simulink model "am_ssb"  (R2014b)
settings: Solver=ode45  StartTime=0.0  StopTime=0.06  RelTol=1e-3
PreLoadFcn:
  | %%%%%%%%%%%%%%%%%%%%%%%%%%%%%%%%%%%%%%%%%%%%%%%%%%%%%%%%%%%%%%%%%%%%%%%%%%%
  | % check to see if Simulink library folder is missing from the MATLAB path %
  | %%%%%%%%%%%%%%%%%%%%%%%%%%%%%%%%%%%%%%%%%%%%%%%%%%%%%%%%%%%%%%%%%%%%%%%%%%%
  | if isempty(strfind(path, 'rtlsdr_book_library'))
  | 
  |     % create error window
  |     fig_error = figure(...
  |         'Name', 'Error: RTL-SDR Book Library',...
  |         'Toolbar','none',...
  |         'MenuBar','none',...
  |         'NumberTitle','off',...
  |         'Resize','off',...
  |         'WindowStyle','modal');
  |     fig_error.Position(3) = 600;
  |     fig_error.Position(4) = 150;
  |     fig_axes = axes(...
  |         'Parent',fig_error,...
  |         'Position',[0,0,1,1],...
  |         'visible','off');
  |     % error message
  |     t_title = text(.05,.8,...
  |         'MISSING DIRECTORIES',...
  |         'FontSize',11.5);
  |     t_body = text(.075,.6,...
  |         [{'Simulink cannot find the  \it{<root>}\rm / \it{rtlsdr\_book\_library}\rm  folder in the \it{MATLAB Path}\rm.'},...
  |         {'Please set the MATLAB path following the instructions given in Exercise 2.4.'}],...
  |         'FontSize',10.5);
  |     % buttons
  |     btn_path = uicontrol(...
  |         'Parent',fig_error,...
  |         'String','Set Path Now',...
  |         'FontSize',10,...
  |         'Callback', 'pathtool; close(fig_error);',...
  |         'Position', [fig_error.Position(3)/2-210, 30, 200, 30]);
  |     btn_abort = uicontrol(...
  |         'Parent',fig_error,...
  |         'String','No thanks',...
  |         'FontSize',10,...
  |         'Callback', 'close(fig_error); abort=1;',...
  |         'Position', [fig_error.Position(3)/2+10, 30, 200, 30]);
  | 
  |     % pause to allow user to interact with error box
  |     uiwait(fig_error);
  | 
  |     % abort simulation
  |     try
  |         if abort==1
  |             set_param(gcs, 'SimulationCommand', 'stop');
  |         end
  |     end
  | 
  |     % if user has set path, allow diagram to be updated
  |     if ~exist('abort','var')
  |         % create error window
  |         fig_update = figure(...
  |             'Name', 'Update Diagram',...
  |             'Toolbar','none',...
  |             'MenuBar','none',...
  |             'NumberTitle','off',...
  |             'Resize','off');
  |         fig_update.Position(3) = 400;
  |         fig_update.Position(4) = 120;
  |         fig_axes = axes(...
  |             'Parent',fig_update,...
  |             'Position',[0,0,1,1],...
  |             'visible','off');
  |         % instruction message
  |         t_body = text(.075,.7,...
  |             'Once you have set the path, update the block diagram',...
  |             'FontSize',10.5);
  |         % button
  |         btn_update = uicontrol(...
  |             'Parent',fig_update,...
  |             'String','Update Block Diagram',...
  |             'FontSize',10,...
  |             'Callback', 'set_param(gcs,''SimulationCommand'',''update''); close(gcf)',...
  |             'Position', [fig_update.Position(3)/2-100, 30, 200, 30]);
  |     end
  | 
  |     % clear error components
  |     clear('fig_error','fig_update','fig_axes','t_title','t_body','btn_path','btn_abort','btn_update','abort');
  | 
  | end
  | %%%%%%%%%%%%%%%%%%%%%%%%%%%%%%%%%%%%%%%%%%%%%%%%%%%%%%%%%%%%%%%%%%%%%%%%%%%
PostLoadFcn:
  | fs  = 200e3;
  | 
  | single.Ai = 8;
  | single.fi = 3e3;
  | single.ph = 0;
  | 
  | bband1.Ai = 1;
  | bband1.fi = 2e3;
  | bband1.ph = pi/2;
  | 
  | bband2.Ai = 3;
  | bband2.fi = 3e3;
  | bband2.ph = 0;
  | 
  | bband3.Ai = 2;
  | bband3.fi = 4e3;
  | bband3.ph = pi/4;
  | 
  | bband4.Ai = 5;
  | bband4.fi = 5e3;
  | bband4.ph = pi/3;
  | 
  | carrier.Ac = 1;
  | carrier.fc = 15e3;
  | carrier.ph = pi/2;
undefined symbols (not defined in the file): fdesignblkfcn, gcbh, startfcn_spectrum_analyzer, startfcn_time_scope
libraries: dspsrcs4 x7, rtlsdr_book_library x1
CloseFcn:
  | closefcn_model;
Description:
  | Software, Simulation Examples and Design Exercises Licence Agreement
  | 
  | This license agreement refers to the simulation examples, design exercises and files,
  | and associated software MATLAB and Simulink resources that accompany the book:
  | 
  |      Title: Software Defined Radio using MATLAB & Simulink and the RTL-SDR
  |      Published by Strathclyde Academic Media, 2015
  |      Authored by Robert W. Stewart, Kenneth W. Barlee, Dale S.W. Atkinson,
  |      and Louise H. Crockett
  | 
  | and made available as a download from, www.desktopSDR.com or variously acquired
  | by other means such as via USB storage, cloud storage, disk or any other electronic
  | or optical or magnetic storage mechanism. These files and associated software may
  | be used subject to the terms of agreement of the conditions below:
  | 
  |     Copyright © 2015 Robert W. Stewart, Kenneth W. Barlee, Dale S.W. Atkinson,
  |     and Louise H. Crockett
  |     All rights reserved.
  | 
  | Redistribution and use in source and binary forms, with or without modification, are
  | permitted provided that the following conditions are met:
  | 
  |    1.  Redistributions of source code must retain the above copyright notice, this list of
  |         conditions and the following disclaimer.
  | 
  |    2.  Redistributions in binary form must reproduce the above copyright notice, this
  |         list of conditions and the following disclaimer in the documentation and/or other
  |         materials provided with the distribution.
  | 
  |    3.  Neither the name of the copyright holder nor the names of its contributors may
  |         be used to endorse or promote products derived from this software without
  |         specific prior written permission.
  | 
  |    4.  In all cases, the software is, and all modifications and derivatives of the
  |         software shall be, licensed to you solely for use in conjunction with The
  |         MathWorks, Inc. products and service offerings.
  | 
  | THIS SOFTWARE IS PROVIDED BY THE COPYRIGHT HOLDERS AND CONTRIBUTORS
  | "AS IS" AND ANY EXPRESS OR IMPLIED WARRANTIES, INCLUDING, BUT NOT LIMITED
  | TO, THE IMPLIED WARRANTIES OF MERCHANTABILITY AND FITNESS FOR A
  | PARTICULAR PURPOSE ARE DISCLAIMED. IN NO EVENT SHALL THE COPYRIGHT
  | HOLDER OR CONTRIBUTORS BE LIABLE FOR ANY DIRECT, INDIRECT, INCIDENTAL,
  | SPECIAL, EXEMPLARY, OR CONSEQUENTIAL DAMAGES (INCLUDING, BUT NOT
  | LIMITED TO, PROCUREMENT OF SUBSTITUTE GOODS OR SERVICES; LOSS OF USE,
  | DATA, OR PROFITS; OR BUSINESS INTERRUPTION) HOWEVER CAUSED AND ON ANY
  | THEORY OF LIABILITY, WHETHER IN CONTRACT, STRICT LIABILITY, OR TORT
  | (INCLUDING NEGLIGENCE OR OTHERWISE) ARISING IN ANY WAY OUT OF THE USE
  | OF THIS SOFTWARE, EVEN IF ADVISED OF THE POSSIBILITY OF SUCH DAMAGE.
  | 
  | 
  | Audio Tracks used in Simulations Examples and Design Exercises
  | 
  | The music and vocal files used within the Examples files and software within the book
  | were variously written, arranged, performed, recorded and produced by Garrey Rice,
  | Adam Struth, Jamie Struth, Iain Thistlethwaite and also Marshall Craigmyle who
  | collectively, and individually where appropriate, assert and retain all of their copyright,
  | performance and artistic rights. Permission to use and reproduce this music is
  | granted for all purposes associated with MATLAB and Simulink software and the
  | simulation examples and design exercises files that accompany this book. Requests to
  | use the music for any other purpose should be directed to: info@desktopSDR.com.
  | For information on music track names, full credits, and links to the musicians please
  | refer to www.desktopSDR.com/more/audio.
settings Model: Creator=desktopSDR Team  LastModifiedBy=desktopSDR Team
settings DataIOCC: LimitDataPoints=off  SaveOutput=off  SignalLogging=off  SaveTime=off

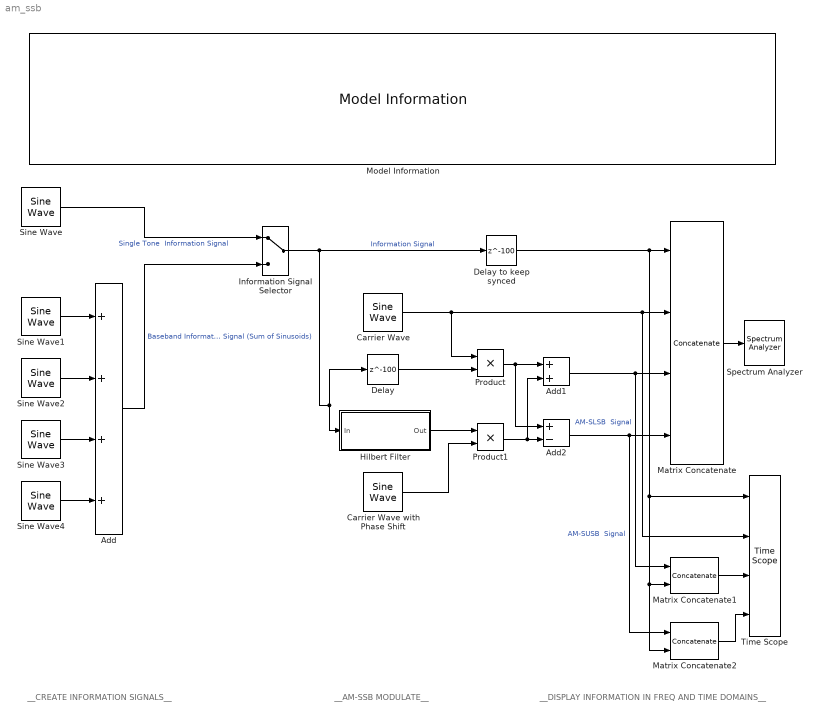
== system am_ssb ==
  note: __CREATE INFORMATION SIGNALS__
  note: __AM-SSB MODULATE__
  note: __DISPLAY INFORMATION IN FREQ AND TIME DOMAINS__
  Add : Sum  Inputs=++++
  Add1 : Sum
  Add2 : Sum  Inputs=+-
  Carrier Wave : dspsrcs4/Sine Wave  Amplitude=carrier.Ac  Frequency=carrier.fc  Phase=carrier.ph  SampleMode=Discrete  OutComplex=Real  CompMethod=Trigonometric fcn  TableSize=Speed  SampleTime=1/fs  SamplesPerFrame=1  ResetState=Restart at time zero  dataType=double  wordLen=16  udDataType=sfix(16)  fracBitsMode=Best precision  numFracBits=15  OutDataTypeStr=double  LastOutDataTypeStr=double
  Carrier Wave with Phase Shift : dspsrcs4/Sine Wave  Amplitude=carrier.Ac  Frequency=carrier.fc  Phase=carrier.ph-(pi/2)  SampleMode=Discrete  OutComplex=Real  CompMethod=Trigonometric fcn  TableSize=Speed  SampleTime=1/fs  SamplesPerFrame=1  ResetState=Restart at time zero  dataType=double  wordLen=16  udDataType=sfix(16)  fracBitsMode=Best precision  numFracBits=15  OutDataTypeStr=double  LastOutDataTypeStr=double
  Delay : Delay  DelayLength=100  InitialCondition=0  InputProcessing=Columns as channels (frame based)
  Delay to keep synced : Delay  DelayLength=100  InitialCondition=0  InputProcessing=Columns as channels (frame based)
  Hilbert Filter : Subsystem  DialogController=fdesignblkfcn  InitFcn=fdesignblkfcn(gcbh, {'InitFcn'});  mask(Hilbert Filter){}
      mask help: Design a Hilbert filter
      settings: CopyFcn=fdesignblkfcn(gcbh, {'CopyFcn'});
      mask Help: helpview(mapfilelocation('dsp'), 'dsphilbertfilter');
      mask Display: disp('Hilbert')
  Information Signal Selector : ManualSwitch
  Matrix Concatenate : Concatenate  NumInputs=4  Mode=Multidimensional array  ConcatenateDimension=2
  Matrix Concatenate1 : Concatenate  Mode=Multidimensional array  ConcatenateDimension=2
  Matrix Concatenate2 : Concatenate  Mode=Multidimensional array  ConcatenateDimension=2
  Model Information : rtlsdr_book_library/Additional Tools/Model Information/Model Information
  Product : Product
  Product1 : Product
  Sine Wave : dspsrcs4/Sine Wave  Amplitude=single.Ai  Frequency=single.fi  Phase=single.ph  SampleMode=Discrete  OutComplex=Real  CompMethod=Trigonometric fcn  TableSize=Speed  SampleTime=1/fs  SamplesPerFrame=1  ResetState=Restart at time zero  dataType=double  wordLen=16  udDataType=sfix(16)  fracBitsMode=Best precision  numFracBits=15  OutDataTypeStr=double  LastOutDataTypeStr=double
  Sine Wave1 : dspsrcs4/Sine Wave  Amplitude=bband1.Ai  Frequency=bband1.fi  Phase=bband1.ph  SampleMode=Discrete  OutComplex=Real  CompMethod=Trigonometric fcn  TableSize=Speed  SampleTime=1/fs  SamplesPerFrame=1  ResetState=Restart at time zero  dataType=double  wordLen=16  udDataType=sfix(16)  fracBitsMode=Best precision  numFracBits=15  OutDataTypeStr=double  LastOutDataTypeStr=double
  Sine Wave2 : dspsrcs4/Sine Wave  Amplitude=bband2.Ai  Frequency=bband2.fi  Phase=bband2.ph  SampleMode=Discrete  OutComplex=Real  CompMethod=Trigonometric fcn  TableSize=Speed  SampleTime=1/fs  SamplesPerFrame=1  ResetState=Restart at time zero  dataType=double  wordLen=16  udDataType=sfix(16)  fracBitsMode=Best precision  numFracBits=15  OutDataTypeStr=double  LastOutDataTypeStr=double
  Sine Wave3 : dspsrcs4/Sine Wave  Amplitude=bband3.Ai  Frequency=bband3.fi  Phase=bband3.ph  SampleMode=Discrete  OutComplex=Real  CompMethod=Trigonometric fcn  TableSize=Speed  SampleTime=1/fs  SamplesPerFrame=1  ResetState=Restart at time zero  dataType=double  wordLen=16  udDataType=sfix(16)  fracBitsMode=Best precision  numFracBits=15  OutDataTypeStr=double  LastOutDataTypeStr=double
  Sine Wave4 : dspsrcs4/Sine Wave  Amplitude=bband4.Ai  Frequency=bband4.fi  Phase=bband4.ph  SampleMode=Discrete  OutComplex=Real  CompMethod=Trigonometric fcn  TableSize=Speed  SampleTime=1/fs  SamplesPerFrame=1  ResetState=Restart at time zero  dataType=double  wordLen=16  udDataType=sfix(16)  fracBitsMode=Best precision  numFracBits=15  OutDataTypeStr=double  LastOutDataTypeStr=double
  Spectrum Analyzer : SpectrumAnalyzer  StartFcn=startfcn_spectrum_analyzer;
  Time Scope : TimeScope  StartFcn=startfcn_time_scope;  DefaultConfigurationName=spbscopes.TimeScopeBlockCfg  NumInputPorts=4
  wires:
  Sine Wave/1 -> Information Signal Selector/1  "Single Tone  Information Signal"
  Add/1 -> Information Signal Selector/2  "Baseband Information Signal (Sum of Sinusoids)"
  Sine Wave1/1 -> Add/1
  Sine Wave2/1 -> Add/2
  Sine Wave4/1 -> Add/4
  Sine Wave3/1 -> Add/3
  Carrier Wave/1 -> Product/1, Time Scope/2, Matrix Concatenate/2
  Matrix Concatenate/1 -> Spectrum Analyzer/1
  Information Signal Selector/1 -> Delay to keep synced/1, Hilbert Filter/1(In), Delay/1  "Information Signal"
  Carrier Wave with Phase Shift/1 -> Product1/2
  Product/1 -> Add2/1, Add1/1
  Product1/1 -> Add2/2, Add1/2
  Add1/1 -> Matrix Concatenate1/1, Matrix Concatenate/3  "AM-SLSB  Signal"
  Add2/1 -> Matrix Concatenate2/1, Matrix Concatenate/4  "AM-SUSB  Signal"
  Matrix Concatenate2/1 -> Time Scope/4
  Delay/1 -> Product/2
  Matrix Concatenate1/1 -> Time Scope/3
  Hilbert Filter/1(Out) -> Product1/1
  Delay to keep synced/1 -> Matrix Concatenate/1, Matrix Concatenate2/2, Matrix Concatenate1/2, Time Scope/1

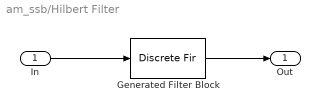
== system am_ssb/Hilbert Filter ==
  In : Inport
  Generated Filter Block : DiscreteFir  Tag=BlockMethodSubSystem  Coefficients=[3.2112005433027521e-16 -8.3766156093897069e-05 2.3614882864187292e-15 -6.5992112024185299e-05 -6.2693327151571844e-16 -9.1525954819870456e-05 -2.0550949302739729e-15 -0.0001231324345604994 -4.5561183535339784e-16 -0.00016173066502508856 1.3219742904112274e-16 -0.00020842367058694102 1.9094108039705036e-15 -0.00026438321164389249 -1.7337676455265223e-15 -0.00033071001178743877 2.6560506310556088e-16 -0.00040869601103557659 3.2724348824688792e-16 -0.00049993156563221501 -1.9389175830615566e-16 -0.00060563845625804993 -2.061570100228298e-15 -0.00072769210664999813 2.3631539552708501e-16 -0.00086767998129710054 -1.1558152391301142e-15 -0.0010274756073035008 -1.6692715976426415e-16 -0.0012090153762096614 -1.4289293336526487e-15 -0.0014144071824742921 -1.4928854039354217e-16 -0.001645847214336256 -1.4202915961995566e-15 -0.0019057282119870761 -3.5775658434049053e-16 -0.0021966459456662021 -2.959233918837667e-15 -0.0025212720850091644 -3.5493113377007693e-16 -0.0028826317064058055 -2.588922546154762e-15 -0.0032838882137399272 2.6140358801167137e-16 -0.0037285693279531795 -2.5993715067853894e-15 -0.0042205296067461123 -3.2363566454187236e-15 -0.0047640841311794579 -8.0007301204506022e-16 -0.0053640296699857815 -1.8009751265730072e-15 -0.0060258227885996163 -2.3963132482591172e-15 -0.0067557074223744407 -2.0734306340991044e-15 -0.0075608679903080567 -3.8935337902945978e-15 -0.0084497865145103934 -8.3845793531854223e-16 -0.0094324724012084249 -2.0759898016990282e-15 -0.010521000368820921 -3.3677428240655131e-15 -0.011730053960380404 -2.8060257732252203e-15 -0.01307780249292817 -1.4790574354314001e-15 -0.014586997591745199 -2.4468204627941198e-15 -0.016286654895417141 -2.2129865523567231e-15 -0.01821438417815191 -2.040951340998615e-15 -0.020419872962853636 -2.1705904925193988e-15 -0.022970237720182363 -2.2009237098912307e-15 -0.025958314811610705 -2.1327375240114386e-15 -0.029516323722934779 -5.8032376500245182e-16 -0.033839039656024195 -2.9979203587109906e-15 -0.039225629524303418 -5.9794403110654907e-16 -0.046159968354213987 -1.9427192351491983e-15 -0.055478713185773687 -1.9854940362495248e-16 -0.068763327967984011 -1.3704745461822756e-15 -0.089404236724447195 -6.7314255523644218e-16 -0.12621888247418989 -5.6810789833163576e-16 -0.21154192368720137 -2.1685200166502347e-16 -0.63639794778019043 0 0.63639794778019043 2.1685200166502347e-16 0.21154192368720137 5.6810789833163576e-16 0.12621888247418989 6.7314255523644218e-16 0.089404236724447195 1.3704745461822756e-15 0.068763327967984011 1.9854940362495248e-16 0.055478713185773687 1.9427192351491983e-15 0.046159968354213987 5.9794403110654907e-16 0.039225629524303418 2.9979203587109906e-15 0.033839039656024195 5.8032376500245182e-16 0.029516323722934779 2.1327375240114386e-15 0.025958314811610705 2.2009237098912307e-15 0.022970237720182363 2.1705904925193988e-15 0.020419872962853636 2.040951340998615e-15 0.01821438417815191 2.2129865523567231e-15 0.016286654895417141 2.4468204627941198e-15 0.014586997591745199 1.4790574354314001e-15 0.01307780249292817 2.8060257732252203e-15 0.011730053960380404 3.3677428240655131e-15 0.010521000368820921 2.0759898016990282e-15 0.0094324724012084249 8.3845793531854223e-16 0.0084497865145103934 3.8935337902945978e-15 0.0075608679903080567 2.0734306340991044e-15 0.0067557074223744407 2.3963132482591172e-15 0.0060258227885996163 1.8009751265730072e-15 0.0053640296699857815 8.0007301204506022e-16 0.0047640841311794579 3.2363566454187236e-15 0.0042205296067461123 2.5993715067853894e-15 0.0037285693279531795 -2.6140358801167137e-16 0.0032838882137399272 2.588922546154762e-15 0.0028826317064058055 3.5493113377007693e-16 0.0025212720850091644 2.959233918837667e-15 0.0021966459456662021 3.5775658434049053e-16 0.0019057282119870761 1.4202915961995566e-15 0.001645847214336256 1.4928854039354217e-16 0.0014144071824742921 1.4289293336526487e-15 0.0012090153762096614 1.6692715976426415e-16 0.0010274756073035008 1.1558152391301142e-15 0.00086767998129710054 ...(+580 chars)]
  Out : Outport
  wires:
  Generated Filter Block/1 -> Out/1
  In/1 -> Generated Filter Block/1
